simulink model "TWAICE_Cell_Model_Farasis_P75_75Ah_v8_1_3"  (R2017b)
settings: Solver=ode3  StartTime=t_start  StopTime=t_end  FixedStep=Ts  RelTol=1e-3
InitFcn:
  | m = Simulink.Mask.get(strcat(model,'/Virtual Battery Tester'));
  | cycler_selection_sel = m.getParameter('cycler_selection');
  | ts_data_repeat_tickbox_sel = m.getParameter('ts_data_repeat_tickbox');
  | if strcmp(cycler_selection_sel.Value, 'Cycle Generator')
  |      t_end = 60*60*24*365*8;
  | elseif strcmp(cycler_selection_sel.Value, 'Timeseries Data')
  |      if strcmp(ts_data_repeat_tickbox_sel.Value, 'off')
  |           t_end = Data.Time(end);
  |      elseif strcmp(ts_data_repeat_tickbox_sel.Value, 'on')
  |            t_end = 60*60*24*365*8;
  |      end
  | end
StartFcn:
  | m = Simulink.Mask.get(strcat(model,'/Virtual Battery Tester'));
  | cycler_selection_sel = m.getParameter('cycler_selection');
  | ts_data_repeat_tickbox_sel = m.getParameter('ts_data_repeat_tickbox');
  | if strcmp(cycler_selection_sel.Value, 'Cycle Generator')
  |      t_end = 60*60*24*365*8;
  | elseif strcmp(cycler_selection_sel.Value, 'Timeseries Data')
  |      if strcmp(ts_data_repeat_tickbox_sel.Value, 'off')
  |           t_end = Data.Time(end);
  |      elseif strcmp(ts_data_repeat_tickbox_sel.Value, 'on')
  |            t_end = 60*60*24*365*8;
  |      end
  | end
model workspace (MAT data in the model file):
  SOC_init = 1
values from neighbouring files (symbols this model uses):
  act = 1    [RunMe_TWAICE_Cell_Model_Farasis_P75_75Ah_v8_1_3.m]
  I_chlim = []    [RunMe_TWAICE_Cell_Model_Farasis_P75_75Ah_v8_1_3.m]
  I_dislim = []    [RunMe_TWAICE_Cell_Model_Farasis_P75_75Ah_v8_1_3.m]
  lic_no = fin_convert(Prod_lic)    [RunMe_TWAICE_Cell_Model_Farasis_P75_75Ah_v8_1_3.m]
  model = 'TWAICE_Cell_Model_Farasis_P75_75Ah_v8_1_3'    [RunMe_TWAICE_Cell_Model_Farasis_P75_75Ah_v8_1_3.m]
  soc_chlim = chargelim.Var2(inx_soc:end)'    [RunMe_TWAICE_Cell_Model_Farasis_P75_75Ah_v8_1_3.m]
  soc_dislim = dischargelim.Var2(inx_soc:end)'    [RunMe_TWAICE_Cell_Model_Farasis_P75_75Ah_v8_1_3.m]
  T_chlim = []    [RunMe_TWAICE_Cell_Model_Farasis_P75_75Ah_v8_1_3.m]
  T_dislim = []    [RunMe_TWAICE_Cell_Model_Farasis_P75_75Ah_v8_1_3.m]
  Ts = 1    [RunMe_TWAICE_Cell_Model_Farasis_P75_75Ah_v8_1_3.m]
undefined symbols (not defined in the file or in its folder): Data, T_init
libraries: simulink x3
(part 1 of 2)
settings Model: Creator=ga56rex  LastModifiedBy=MATLAB-Compute2
settings DataIOCC: LimitDataPoints=on  SaveFormat=StructureWithTime  ReturnWorkspaceOutputs=on
settings OptimizationCC: BlockReduction=off  BooleanDataType=off
settings DebuggingCC: ReadBeforeWriteMsg=DisableAll  WriteAfterWriteMsg=DisableAll  WriteAfterReadMsg=DisableAll  AlgebraicLoopMsg=error  SaveWithParameterizedLinksMsg=none  InheritedTsInSrcMsg=none  AllowSymbolicDim=off  StrictBusMsg=ErrorOnBusTreatedAsVector  SFUnexpectedBacktrackingDiag=warning  SFNoUnconditionalDefaultTransitionDiag=warning  SFExecutionAtInitializationDiag=none
settings HardwareCC: ProdBitPerPointer=32  ProdBitPerSizeT=32  ProdBitPerPtrDiffT=32  ProdLargestAtomicFloat=None  ProdIntDivRoundTo=Undefined  ProdEndianess=Unspecified  ProdWordSize=32  ProdHWDeviceType=32-bit Generic  TargetBitPerPointer=64  TargetBitPerSizeT=64  TargetBitPerPtrDiffT=64  TargetLongLongMode=on  TargetIntDivRoundTo=Zero  TargetEndianess=LittleEndian  TargetWordSize=64  TargetHWDeviceType=MATLAB Host  ProdEqTarget=off
settings ModelReferenceCC: PropagateSignalLabelsOutOfModel=off  SupportModelReferenceSimTargetCustomCode=on
settings SFSimCC: SimUserLibraries=LexActivator.lib  SimParseCustomCode=off
settings SFSimCC: SimCustomHeaderCode=|
  | #include "LexActivator.h"
  | #include "LexStatusCodes.h"
settings RTWCC: SystemTargetFile=rtwsfcn.tlc  TemplateMakefile=rtwsfcn_default_tmf  Description=S-Function Target  RTWUseSimCustomCode=on  CustomLibrary=LexActivator.lib
settings RTWCC: CustomHeaderCode=|
  | #include "LexActivator.h"
  | #include "LexStatusCodes.h"
settings CodeAppCC: StateflowObjectComments=on
settings STFCustomTargetCC: ModelReferenceCompliant=off  CompOptLevelCompliant=on  MATLABClassNameForMDSCustomization=Simulink.SoftwareTarget.TargetSpecificTriggerConfigurationBase  SystemTargetFile=rtwsfcn.tlc
settings ConfigComp: CovMetricSettings=dw  CovSaveCumulativeToWorkspaceVar=on  CovSaveSingleToWorkspaceVar=on  CovExternalEMLEnable=off  CovSFcnEnable=off

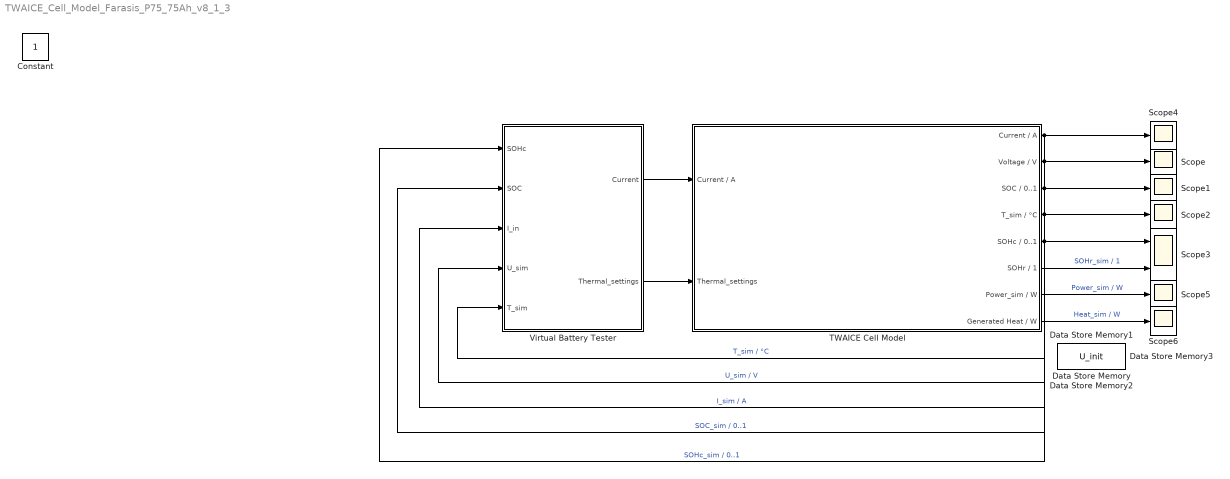
== system TWAICE_Cell_Model_Farasis_P75_75Ah_v8_1_3 ==
  Data Store Memory : DataStoreMemory  DataStoreName=SOHc_init  ReadBeforeWriteMsg=warning  WriteAfterWriteMsg=warning  WriteAfterReadMsg=warning  ShowAdditionalParam=off
  Data Store Memory1 : DataStoreMemory  DataStoreName=SOC_init  ReadBeforeWriteMsg=warning  WriteAfterWriteMsg=warning  WriteAfterReadMsg=warning  ShowAdditionalParam=off
  Data Store Memory2 : DataStoreMemory  DataStoreName=T_init  ReadBeforeWriteMsg=warning  WriteAfterWriteMsg=warning  WriteAfterReadMsg=warning  ShowAdditionalParam=off
  Data Store Memory3 : DataStoreMemory  DataStoreName=U_init  ReadBeforeWriteMsg=warning  WriteAfterWriteMsg=warning  WriteAfterReadMsg=warning  ShowAdditionalParam=off
  Scope{,1..2,4..6} (6 alike) : Scope
  Scope3 : Scope  NumInputPorts=2
  TWAICE Cell Model : Subsystem  mask{SOHc_init=1.0, SOHr_init=1.0, T_init=25, SOC_init=0.5}
      mask prompts: SOHc_init "SOHc / 0..1"; SOHr_init "SOHr / 1"; T_init "T_cell / °C"; SOC_init "SOC / 0..1"
      mask init:
      | %set_param('TWAICE_Cell_Model_MANUFACTURER_CELLTYPE_v4_2_open/TWAICE CELL MODEL','backgroundcolor','[1 0 1]')
      mask DialogControl Control4 Prompt: Electric-Thermal-Aging Model
      mask DialogControl DescTextVar Prompt: Setting Initial Parameters for the Model
      mask DialogControl Container11 Prompt: Aging
      mask DialogControl Container13 Prompt: Electric and Thermal
      mask Display: image('config/TwaiceCellModel.png'); % Use "Edit Image" on toolstrip to change.
  Virtual Battery Tester : Subsystem  mask{cycler_selection=Cycle Generator, trigger_current_ch=on, value_profile_ch=50, trigger_power_ch=off, value_charge_pause=60, discharge_type=Constant, trigger_current_dis=on, value_profile_dis=75, trigger_power_dis=off, value_discharge_pause=60, trigger_depth_dis_soc=on, value_depth_dis_soc=0, trigger_depth_dis_U=off, value_depth_dis_U=3, trigger_cv_discharge=off, value_cv_discharge_stop=0, trigger_depth_ch_soc=on, value_depth_ch_soc=1, trigger_depth_ch_U=off, value_depth_ch_U=4.2, trigger_cv_charge=off, value_cv_charge_stop=0, trigger_custom_part_resting=off, value_resting_soc=0.3, value_repeating_cycles=1, value_resting_time=20000, T_amb_set=25, stop_parameter=Equivalent Full Cycles / -, stop_value=50, start_condition=Charge, default_thermal_settings_cycgen=Use default fitted parameters, value_htc_cycgen=NaN, value_Pcool_cycgen=NaN, ts_data_profile_selection=Current / A, ts_data_repeat_tickbox=off, stop_parameter_ts_data=SOHc / 1...0, stop_value_ts_data=0.8, default_thermal_settings_ts_data=Use default fitted parameters, value_htc_ts_data=NaN, value_Pcool_ts_data=NaN, controller_tickbox=off, ctrl_type=SOC / 0...1, lower_bound_voltage=2.2, upper_bound_voltage=4.5, lower_bound_soc=0, upper_bound_soc=1, violation_trigger=off, trigger_chargelim=off, trigger_dischargelim=off}
      mask prompts: trigger_current_ch "Current / A"; value_profile_ch "Constant"; trigger_power_ch "Power / W"; value_charge_pause "Pause After Charge / s"; trigger_current_dis "Current / A"; value_profile_dis "Constant"; trigger_power_dis "Power / W"; value_discharge_pause "Pause After Discharge / s"; trigger_depth_dis_soc "SOC / 0...1"; value_depth_dis_soc "0 to 1"; trigger_depth_dis_U "Voltage / V"; trigger_cv_discharge "CV Cutoff Current Discharge/ A"; trigger_depth_ch_soc "SOC / 0...1"; value_depth_ch_soc "0 to 1"; trigger_depth_ch_U "Voltage / V"; trigger_cv_charge "CV Cutoff Current Charge / A"; trigger_custom_part_resting "Enable rest at defined SOC during cycling"; value_resting_soc "Resting SOC / 0...1"; value_repeating_cycles "Number of repeating cycles / -"; value_resting_time "Resting time / s"; ts_data_profile_selection "Input Profile"; ts_data_repeat_tickbox "Repeat timeseries data input and apply manually selected stop criteria."; controller_tickbox "Apply global cell limits"; ctrl_type "Type"; lower_bound_voltage "Global minimum voltage / V"; upper_bound_voltage "Global maximum voltage / V"; lower_bound_soc "Lower boundary SOC / 0...1"; upper_bound_soc "Upper boundary SOC / 0...1"; violation_trigger "Stop simulation upon violation (for unchecked box simulation continues with current set to zero outside the specified boundaries)"; trigger_chargelim "Enable current limitation during charging"; trigger_dischargelim "Enable current limitation during discharging"
      mask init:
      | if start_condition == 1
      |     u1_init = 0;
      | elseif start_condition == 2
      |     u1_init = 3;
      | end
      | 
      | %% Current or Power Charging
      | m = Simulink.Mask.get(gcb);
      | box_A = get_param(gcb, 'trigger_current_ch');
      | box_B = m.getParameter('trigger_power_ch');
      | if strcmp(box_A, 'off') &&  strcmp(box_B, 'off')
      |     u1_init = 10;
      | end
      mask Help:
      | This Tool generates a synthetic Power/Current Profile within specified Voltage or SOC Boundaries.
      | 
      | Box Profile Charge: Either current or power. Ticking both applies a current profile as default value.
      | 
      | Box Profile Discharge: Either current or power. Ticking both applies a current profile as default value.
      | 
      | Profile from Workspace: uses user profile in discharge direction. Must be loaded to workspace in format timeseries and named "Data_Discharge". Make sure the Data is not cleared at simulation start or reloaded into workspace. Timeseries Data must consist of the time and current/power data. Generate with: Data_Discharge = timeseries(Data, time);
      | 
      | Cycle Depth: Stop Charge/Discharge either at specified SOC or Voltage. Ticking both uses SOC as default value. SOC ranges from 0 to 1. CV phase only possible when specifying Voltage as Stop Criteria.
      | 
      | Start Condition: Charge or Discharge.
      | 
      | Stop Condition: EFC, Cycles, Time or SOHc (Capacity)
      mask TypeOptions cycler_selection: Cycle Generator | Timeseries Data
      mask Callback cycler_selection:
      | %%
      | % Enable Disable Cycle Generator and Timeseries Data Tab
      | % Block to be used modular
      | %msk_vbt = Simulink.Mask.get(strcat(model,'/Virtual Battery Tester'));
      | msk_vbt = Simulink.Mask.get(gcb);
      | for i = 1:length(msk_vbt.Parameters)
      |     names_vbt_mask{i,1} = msk_vbt.Parameters(i).Name;
      | end
      | 
      | % Block only here used
      | box_tickbox = get_param(gcb, 'cycler_selection');
      | inx_cyclegenerator_block_start = find(contains(names_vbt_mask,...
      |         'trigger_current_ch'));
      | inx_cyclegenerator_custom_part_resting = find(contains(names_vbt_mask,...
      |         'trigger_custom_part_resting'));
      | inx_cyclegenerator_T_amb = find(contains(names_vbt_mask,...
      |         'T_amb_set'));
      | inx_cyclegenerator_default_thermal_settings = find(contains(names_vbt_mask,...
      |         'default_thermal_settings_cycgen'));
      | 
      | 
      | inx_timeseriesdata_block_start = find(contains(names_vbt_mask,...
      |         'ts_data_profile_selection'));
      | inx_timeseriesdata_stop_criteria = find(contains(names_vbt_mask,...
      |         'ts_data_repeat_tickbox'));
      | inx_timeseriesdata_default_thermal_settings_ts_data = find(contains(names_vbt_mask,...
      |         'default_thermal_settings_ts_data'));
      | inx_batterycontroller_block_start = find(contains(names_vbt_mask,...
      |         'controller_tickbox'));
      | 
      | if strcmp(box_tickbox, 'Cycle Generator')
      |     % Enable Cycle Generator Block from Start to Enable Resting SOC
      |     for i_mask = inx_cyclegenerator_block_start:inx_cyclegenerator_custom_part_resting
      |         msk_vbt.Parameters(1,i_mask).Enabled = 'on';
      |     end
      |     for i_mask = inx_cyclegenerator_T_amb:inx_cyclegenerator_default_thermal_settings
      |         % Enable Cycle Generator Block from T_ambient to Radio Button
      |         % Default Thermal Setting but Default values yet as disabled
      |         msk_vbt.Parameters(1,i_mask).Enabled = 'on';
      |     end
      |     % Disable Timeseries Data Block
      |     for i_mask = inx_timeseriesdata_block_start:inx_batterycontroller_block_start-1
      |         msk_vbt.Parameters(1,i_mask).Enabled = 'off';
      |     end
      |     msk_vbt.Parameters(1,inx_timeseriesdata_stop_criteria).Value = 'off'; % Set TS Data Stop Criteria to Off (in addition to disabled)
      |     msk_vbt.Parameters(1,inx_timeseriesdata_default_thermal_settings_ts_data).Value = 'Use default fitted parameters'; % Set Thermal Parameters Ts Data to Default (in addition to disabled)
      | elseif strcmp(box_tickbox, 'Timeseries Data')
      |     for i_mask = inx_cyclegenerator_block_start:inx_timeseriesdata_block_start-1
      |         % Disable Cycle Generator Block
      |         msk_vbt.Parameters(1,i_mask).Enabled = 'off';
      |     end
      |     msk_vbt.Parameters(1,inx_cyclegenerator_custom_part_resting).Value = 'off'; % Set Enable Resting to Off (in addition to disabled)
      |     msk_vbt.Parameters(1,inx_cyclegenerator_default_thermal_settings).Value = 'Use default fitted parameters'; % Set Thermal Parameters Cyc Gen to Default (in addition to disabled)
      | 
      |     for i_mask = inx_timeseriesdata_block_start:inx_timeseriesdata_stop_criteria
      |         % Enable Timeseries Data Block
      |         msk_vbt.Parameters(1,i_mask).Enabled = 'on';
      |     end
      |     for i_mask = inx_timeseriesdata_default_thermal_settings_ts_data
      |         % Enable Timeseries Data Block
      |         msk_vbt.Parameters(1,i_mask).Enabled = 'on';
      |     end
      | end
      mask Callback trigger_current_ch:
      | %% Current or Power Charging
      | m = Simulink.Mask.get(gcb);
      | box_A = get_param(gcb, 'trigger_current_ch');
      | box_B = m.getParameter('trigger_power_ch');
      | if strcmp(box_A, 'on')
      |     box_B.Value = 'off';
      | end
      mask Callback trigger_power_ch:
      | %% Current or Power Charging
      | m = Simulink.Mask.get(gcb);
      | box_A = m.getParameter( 'trigger_current_ch');
      | box_B = get_param(gcb, 'trigger_power_ch');
      | if strcmp(box_B, 'on')
      |     box_A.Value = 'off';
      | end
      mask TypeOptions discharge_type: Constant | Profile from Workspace (Name in Workspace: Data_Discharge)
      mask Callback discharge_type:
      | m = Simulink.Mask.get(gcb);
      | dis_type = m.getParameter('discharge_type');
      | box_dis_value = m.getParameter('value_profile_dis');
      | if strcmp(dis_type.Value, 'Profile from Workspace (Name in Workspace: Data_Discharge)')
      |     box_dis_value.Enabled = 'off';
      | elseif strcmp(dis_type.Value, 'Constant')
      |     box_dis_value.Enabled = 'on';
      | end
      mask Callback trigger_current_dis:
      | %% Current or Power Discharging
      | m = Simulink.Mask.get(gcb);
      | box_A = get_param(gcb, 'trigger_current_dis');
      | box_B = m.getParameter('trigger_power_dis');
      | if strcmp(box_A, 'on')
      |     box_B.Value = 'off';
      | end
      mask Callback trigger_power_dis:
      | %% Current or Power Charging
      | m = Simulink.Mask.get(gcb);
      | box_A = m.getParameter( 'trigger_current_dis');
      | box_B = get_param(gcb, 'trigger_power_dis');
      | if strcmp(box_B, 'on')
      |     box_A.Value = 'off';
      | end
      mask Callback trigger_depth_dis_soc:
      | m = Simulink.Mask.get(gcb);
      | box_soc = get_param(gcb, 'trigger_depth_dis_soc');
      | box_U = m.getParameter('trigger_depth_dis_U');
      | box_CV = m.getParameter('trigger_cv_discharge');
      | box_CVvalue = m.getParameter('value_cv_discharge_stop');
      | if strcmp(box_soc, 'on')
      |     box_U.Value = 'off';
      |     box_CV.Value = 'off';
      |     box_CV.Enabled = 'off';
      |     box_CVvalue.Enabled = 'off';
      | end
      mask Callback trigger_depth_dis_U:
      | m = Simulink.Mask.get(gcb);
      | box_soc = m.getParameter( 'trigger_depth_dis_soc');
      | box_U = get_param(gcb,'trigger_depth_dis_U');
      | box_CV = m.getParameter('trigger_cv_discharge');
      | box_CVvalue = m.getParameter('value_cv_discharge_stop');
      | if strcmp(box_U, 'on')
      |     box_soc.Value = 'off';
      |     box_CVvalue.Enabled = 'on';
      |     box_CV.Enabled = 'on';
      | end
      mask Callback trigger_depth_ch_soc:
      | m = Simulink.Mask.get(gcb);
      | box_soc = get_param(gcb, 'trigger_depth_ch_soc');
      | box_U = m.getParameter('trigger_depth_ch_U');
      | box_CV = m.getParameter('trigger_cv_charge');
      | box_CVvalue = m.getParameter('value_cv_charge_stop');
      | if strcmp(box_soc, 'on')
      |     box_U.Value = 'off';
      |     box_CV.Value = 'off';
      |     box_CV.Enabled = 'off';
      |     box_CVvalue.Enabled = 'off';
      | end
      mask Callback trigger_depth_ch_U:
      | m = Simulink.Mask.get(gcb);
      | box_soc = m.getParameter( 'trigger_depth_ch_soc');
      | box_U = get_param(gcb,'trigger_depth_ch_U');
      | box_CV = m.getParameter('trigger_cv_charge');
      | box_CVvalue = m.getParameter('value_cv_charge_stop');
      | if strcmp(box_U, 'on')
      |     box_soc.Value = 'off';
      |     box_CVvalue.Enabled = 'on';
      |     box_CV.Enabled = 'on';
      | end
      mask Callback trigger_custom_part_resting:
      | %% Current or Power Charging
      | m = Simulink.Mask.get(gcb);
      | tickbox_custom_part_fluence = get_param(gcb, 'trigger_custom_part_resting');
      | box_rep_cycles = m.getParameter('value_repeating_cycles');
      | box_rest_time = m.getParameter('value_resting_time');
      | box_rest_soc = m.getParameter('value_resting_soc');
      | if strcmp(tickbox_custom_part_fluence, 'off')
      |     box_rep_cycles.Enabled = 'off';
      |     box_rest_time.Enabled = 'off';
      |     box_rest_soc.Enabled = 'off';
      | elseif strcmp(tickbox_custom_part_fluence, 'on')
      |     box_rep_cycles.Enabled = 'on';
      |     box_rest_time.Enabled = 'on';
      |     box_rest_soc.Enabled = 'on';
      | end
      mask TypeOptions stop_parameter: Equivalent Full Cycles / - | Cycles / - | Time / h | SOHc / 1...0
      mask TypeOptions start_condition: Charge | Discharge
      mask TypeOptions default_thermal_settings_cycgen: Use default fitted parameters | Use own adjustable parameters
      mask Callback default_thermal_settings_cycgen:
      | % Enable Disable Thermal Parameter Usage Cycle Generator
      | % Block to be used modular
      | msk_thermal_set_cycgen = Simulink.Mask.get(gcb);
      | for i = 1:length(msk_thermal_set_cycgen.Parameters)
      |     names_vbt_mask{i,1} = msk_thermal_set_cycgen.Parameters(i).Name;
      | end
      | 
      | inx_thermal_setting_cyc_generator_start = find(contains(names_vbt_mask,...
      |         'value_htc_cycgen'));
      | inx_thermal_setting_cyc_generator_end = find(contains(names_vbt_mask,...
      |         'value_Pcool_cycgen'));
      | box_thermalsetings_cycgen = get_param(gcb, 'default_thermal_settings_cycgen');
      | 
      | if strcmp(box_thermalsetings_cycgen, 'Use default fitted parameters')
      |     for i_mask = inx_thermal_setting_cyc_generator_start:inx_thermal_setting_cyc_generator_end
      |         % Disable adjustable parameters
      |         msk_thermal_set_cycgen.Parameters(1,i_mask).Enabled = 'off';
      |     end
      | elseif strcmp(box_thermalsetings_cycgen, 'Use own adjustable parameters')
      |     for i_mask = inx_thermal_setting_cyc_generator_start:inx_thermal_setting_cyc_generator_end
      |         % Enable adjustable parameters
      |         msk_thermal_set_cycgen.Parameters(1,i_mask).Enabled = 'on';
      |     end
      | end
      mask TypeOptions ts_data_profile_selection: Current / A | Power / W
      mask Callback ts_data_repeat_tickbox:
      | m = Simulink.Mask.get(gcb);
      | box_tickbox = get_param(gcb, 'ts_data_repeat_tickbox');
      | box_stop = m.getParameter('stop_parameter_ts_data');
      | box_stop2 = m.getParameter('stop_value_ts_data');
      | if strcmp(box_tickbox, 'on')
      |     box_stop.Enabled = 'on';
      |     box_stop2.Enabled = 'on';
      | end
      | if strcmp(box_tickbox, 'off')
      |     box_stop.Enabled = 'off';
      |     box_stop2.Enabled = 'off';
      | end
      mask TypeOptions stop_parameter_ts_data: Equivalent Full Cycles / - | Time / h | SOHc / 1...0
      mask TypeOptions default_thermal_settings_ts_data: Use default fitted parameters | Use own adjustable parameters
      mask Callback default_thermal_settings_ts_data:
      | % Enable Disable Thermal Parameter Usage Timeseries Data
      | % Block to be used modular
      | msk_thermal_set_ts_data = Simulink.Mask.get(gcb);
      | for i = 1:length(msk_thermal_set_ts_data.Parameters)
      |     names_vbt_mask{i,1} = msk_thermal_set_ts_data.Parameters(i).Name;
      | end
      | 
      | inx_thermal_setting_ts_data_start = find(contains(names_vbt_mask,...
      |         'value_htc_ts_data'));
      | inx_thermal_setting_ts_data_end = find(contains(names_vbt_mask,...
      |         'value_Pcool_ts_data'));
      | box_thermalsetings_ts_data = get_param(gcb, 'default_thermal_settings_ts_data');
      | 
      | if strcmp(box_thermalsetings_ts_data, 'Use default fitted parameters')
      |     for i_mask = inx_thermal_setting_ts_data_start:inx_thermal_setting_ts_data_end
      |         % Disable adjustable parameters
      |         msk_thermal_set_ts_data.Parameters(1,i_mask).Enabled = 'off';
      |     end
      | elseif strcmp(box_thermalsetings_ts_data, 'Use own adjustable parameters')
      |     for i_mask = inx_thermal_setting_ts_data_start:inx_thermal_setting_ts_data_end
      |         % Enable adjustable parameters
      |         msk_thermal_set_ts_data.Parameters(1,i_mask).Enabled = 'on';
      |     end
      | end
      mask Callback controller_tickbox:
      | m = Simulink.Mask.get(gcb);
      | box_controller = get_param(gcb, 'controller_tickbox');
      | box_1 = m.getParameter('ctrl_type');
      | box_2 = m.getParameter('lower_bound_voltage');
      | box_3 = m.getParameter('upper_bound_voltage');
      | box_4 = m.getParameter('lower_bound_soc');
      | box_5 = m.getParameter('upper_bound_soc');
      | box_6 = m.getParameter('violation_trigger');
      | box_7 = m.getParameter('trigger_chargelim');
      | box_8 = m.getParameter('trigger_dischargelim');
      | if strcmp(box_controller, 'off')
      |     box_1.Enabled = 'off';
      |     box_2.Enabled = 'off';
      |     box_3.Enabled = 'off';
      |     box_4.Enabled = 'off';
      |     box_5.Enabled = 'off';
      |     box_6.Enabled = 'off';
      |     box_7.Enabled = 'off';
      |     box_8.Enabled = 'off';
      | elseif strcmp(box_controller, 'on')
      |     box_1.Enabled = 'on';
      |     box_2.Enabled = 'on';
      |     box_3.Enabled = 'on';
      |     box_4.Enabled = 'on';
      |     box_5.Enabled = 'on';
      |     box_6.Enabled = 'on';
      |     box_7.Enabled = 'on';
      |     box_8.Enabled = 'on';
      | end
      mask TypeOptions ctrl_type: Voltage / V | SOC / 0...1
      mask Callback ctrl_type:
      | %% Current or Power Charging
      | m = Simulink.Mask.get(gcb);
      | box_type = get_param(gcb, 'ctrl_type');
      | box_min_voltage = m.getParameter( 'lower_bound_voltage');
      | box_max_voltage = m.getParameter( 'upper_bound_voltage');
      | box_min_soc = m.getParameter('lower_bound_soc');
      | box_max_soc = m.getParameter( 'upper_bound_soc');
      | 
      | if strcmp(box_type, 'Voltage / V')
      |      box_min_soc.Enabled = 'off';
      |      box_max_soc.Enabled = 'off';
      |      box_min_voltage.Enabled = 'on';
      |      box_max_voltage.Enabled = 'on';
      |  elseif strcmp(box_type, 'SOC / 0...1')
      |     box_min_soc.Enabled = 'on';
      |     box_max_soc.Enabled = 'on';
      |     box_min_voltage.Enabled = 'off';
      |     box_max_voltage.Enabled = 'off';
      |  end
      mask DialogControl Control7 Prompt: With this interface virtual battery testing is performed. Either a cycle generator can be used to generate synthetic profiles consisting of constant charge and discharge conditions within specified limits. Alternatively, timeseries data (current or power and ambient temperature) from the MATLAB workspace can be used as input into the TWAICE cell model
      mask DialogControl Container39 Prompt: Main Selection
      mask DialogControl Control41 Prompt: Use only Cycle Generator OR Timeseries Data. Please do not use both.
      mask DialogControl Control42 Prompt: Please select one of the following:
      mask DialogControl cyc_gen_container Prompt: Cycle Generator
      mask DialogControl Current_Power Prompt: Cycle Generator Options
      mask DialogControl Control38 Prompt: With the cycle generator virtual charge, discharge cycles with constant conditions can be selected.
      mask DialogControl Control39 Prompt: The constant current or power values and the upper and lower boundaries can be selected.
      mask DialogControl ChargeProfile Prompt: Charge
      mask DialogControl DischargeProfile Prompt: Discharge
      mask DialogControl Control23 Prompt: For discharge a constant value or timeseries data from the workspace can be used.
      mask DialogControl Control24 Prompt: The discharge data must be named Data_Discharge in the MATLAB workspace with the following format:
      mask DialogControl Control28 Prompt: Data_Discharge = timeseries(I, t) or Data_Discharge = timeseries(P, t) with
      mask DialogControl Control25 Prompt: - Time t in seconds
      mask DialogControl Control26 Prompt: - Current I in Ampere or Power P in W
      mask DialogControl Cycle_Depth Prompt: Cycle Depth
      mask DialogControl DischargeProfile_copy Prompt: Stop Discharge At
      mask DialogControl ChargeDepth Prompt: Stop Charge At
      mask DialogControl Rest_phase_extension Prompt: Rest at defined SOC during cycling
      mask DialogControl Control47 Prompt: With this feature, resting phases can be introduced during cycling. Before each pause, the cell will be charged to and hold at a resting SOC. At the end of the pause, the cell will be charged to the defined upper limit. Tunable parameters are:
      mask DialogControl Control48 Prompt: - Resting SOC: SOC, at which the cell should be held. Resting SOC must be above the discharge stop condition.
      mask DialogControl Control49 Prompt: - Number of repeating cycles: number of cycles to be repeated before going into the resting phase.
      mask DialogControl Control50 Prompt: - Resting time: duration of the resting period in seconds before charging to the upper limit.
      mask DialogControl Control15 Prompt: Ambient Temperature /  °C
      mask DialogControl Container10 Prompt: Start and Stop Condition
      mask DialogControl Container17 Prompt: Stop Condition
      mask DialogControl Container14 Prompt: Start Condition
      mask DialogControl Container43 Prompt: Thermal settings Cycle Generator
      mask DialogControl txt_htc Prompt: Convective heat transfer coefficient / W/(Km^2)
      mask DialogControl txt_Pcool Prompt: Cooling (>0) or heating (<0) power / W
      mask DialogControl ts_data_container Prompt: Timeseries Data
      mask DialogControl Container42 Prompt: Timeseries Data Options
      mask DialogControl Control16 Prompt: With this option the cell behaviour is simulated for timeseries data from the workspace.
      mask DialogControl Control17 Prompt: The data must be named Data in the MATLAB workspace with the following format:
      mask DialogControl Control19 Prompt: Data = timeseries([I, T_amb] , t) or Data = timeseries([P, T_amb], t) with
      mask DialogControl Control20 Prompt: - Time t in seconds.
      mask DialogControl Control21 Prompt: - Current I in Ampere or Power P in Watt.
      mask DialogControl Control31 Prompt: - Ambient Temperature T_amb in °C.
      mask DialogControl Container10_copy Prompt: Stop Condition
      mask DialogControl Control33 Prompt: By default the simulation stops once the input timeseries data ends.
      mask DialogControl Control34 Prompt: Alternatively, in this section it can be selected to repeat the input data until reaching a user defined stop criteria.
      mask DialogControl Container_ts_data Prompt: Stop Condition
      mask DialogControl Container44 Prompt: Thermal settings Timeseries Data
      mask DialogControl txt_htc_ts_data Prompt: Convective heat transfer coefficient / W/(Km^2)
      mask DialogControl txt_Pcool_ts_data Prompt: Cooling (>0) or heating (<0) power / W
      mask DialogControl Container38 Prompt: Battery Controller
      mask DialogControl Control8 Prompt: With this Controller, global voltage, SOC and temperature limits can be specified. Outside these specified boundaries the current is automatically set to zero. This battery controller can be enabled for both options (Cycle Generator and Timeseries Data).
      mask DialogControl Container31 Prompt: Global SOC/voltage limits
      mask DialogControl Control10 Prompt: Reaching those limits the current is set to zero or the simulation stopped depending on user selection.
      mask DialogControl Container32 Prompt: Current limits in dependency of temperature and SOC
      mask DialogControl Control13 Prompt: Enable maximum current limits as function of cell temperature and SOC. These can be entered seperately for charging and discharging in the excel:
      mask DialogControl Control14 Prompt: T_SOC_based_CurrentLimits.xlsx
      mask DialogControl Control14 Callback: winopen('./config/T_SOC_based_CurrentLimits.xlsx')
      mask DialogControl Control37 Prompt: Info: After changes, excel must be saved and RunMe file must be re-run to load in the latest changes into the MATLAB workspace.
      mask Display: image('config/VirtualBatteryTester.PNG'); % Use "Edit Image" on toolstrip to change.
  Constant : Constant  IOType=siggen
  wires:
  TWAICE Cell Model/3(SOC / 0..1) -> Virtual Battery Tester/2(SOC), Scope1/1  "SOC_sim / 0..1"
  TWAICE Cell Model/8(Generated Heat / W) -> Scope6/1  "Heat_sim / W"
  TWAICE Cell Model/7(Power_sim / W) -> Scope5/1  "Power_sim / W"
  TWAICE Cell Model/2(Voltage / V) -> Virtual Battery Tester/4(U_sim), Scope/1  "U_sim / V"
  TWAICE Cell Model/1(Current / A) -> Scope4/1, Virtual Battery Tester/3(I_in)  "I_sim / A"
  TWAICE Cell Model/4(T_sim / °C) -> Virtual Battery Tester/5(T_sim), Scope2/1  "T_sim / °C"
  TWAICE Cell Model/5(SOHc / 0..1) -> Virtual Battery Tester/1(SOHc), Scope3/1  "SOHc_sim / 0..1"
  TWAICE Cell Model/6(SOHr / 1) -> Scope3/2  "SOHr_sim / 1"
  Virtual Battery Tester/1(Current) -> TWAICE Cell Model/1("Current / A ")
  Virtual Battery Tester/2(Thermal_settings) -> TWAICE Cell Model/2(Thermal_settings)

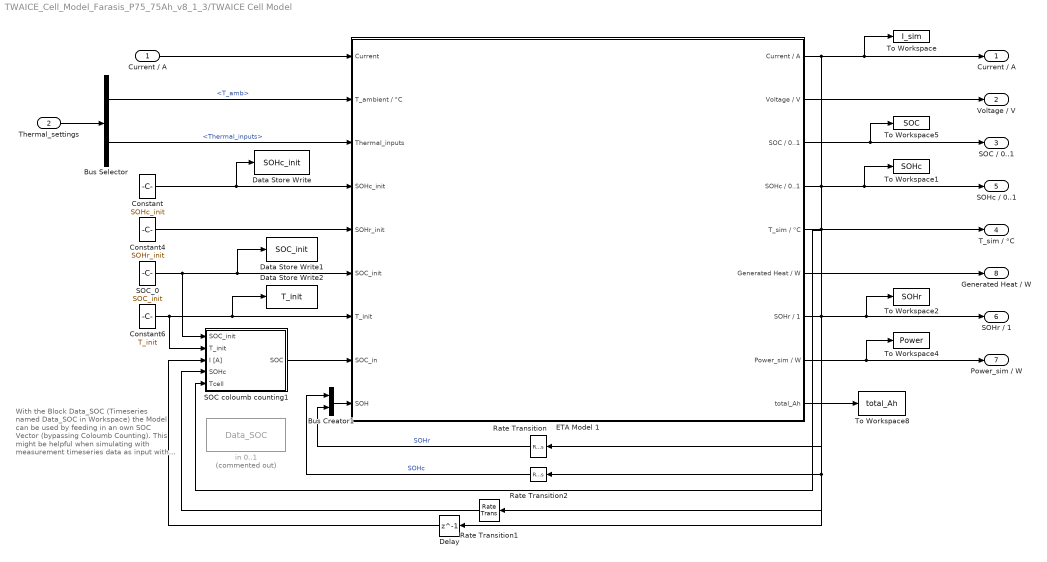
== system TWAICE_Cell_Model_Farasis_P75_75Ah_v8_1_3/TWAICE Cell Model ==
  note: With the Block Data_SOC (Timeseries named Data_SOC in Workspace)  the Model can be used by feeding in an own SOC Vector (bypassing Coloumb Counting). This might be helpful when simulating with measurement timeseries data as input with a strong SOC drift during coloumb counting.
      | For this the Block Data_SOC is to be uncommented and connected with the input SOC_in into the ETA Model.
  "Current / A " : Inport  OutDataTypeStr=double  PortDimensions=1
  Thermal_settings : Inport  Port=2
  Bus Creator1 : BusCreator  Inputs=2
  Bus Selector : BusSelector  OutputSignals=T_amb,Thermal_inputs
  Constant : Constant  Value=SOHc_init
  Constant4 : Constant  Value=SOHr_init
  Constant6 : Constant  Value=T_init
  Data Store Write : DataStoreWrite  DataStoreName=SOHc_init
  Data Store Write1 : DataStoreWrite  DataStoreName=SOC_init
  Data Store Write2 : DataStoreWrite  DataStoreName=T_init
  Delay : Delay  DelayLength=1
  ETA Model 1 : Subsystem  mask{sfcnParam1=Ts, sfcnParam2=act, sfcnParam3=lic_no}
      mask prompts: sfcnParam1 "Ts:"; sfcnParam2 "act:"; sfcnParam3 "lic_no:"
      mask help: Simulink:masks:GenSFuncDesc_MD
      mask Help: eval('feval(''rtwprivate'',''rtwhelpview'',''rtw_sfcn_block'')');
  Rate Transition : RateTransition  InitialCondition=SOHr_init
  Rate Transition1 : RateTransition  InitialCondition=SOHc_init
  Rate Transition2 : RateTransition  InitialCondition=SOHc_init
  SOC coloumb counting1 : Subsystem  mask{sfcnParam1=Ts}
      mask prompts: sfcnParam1 "Ts:"
      mask help: Simulink:masks:GenSFuncDesc_MD
      mask Help: eval('feval(''rtwprivate'',''rtwhelpview'',''rtw_sfcn_block'')');
  SOC_0 : Constant  Value=SOC_init
  To Workspace : ToWorkspace  VariableName=I_sim  SaveFormat=Timeseries  SampleTime=-1
  To Workspace1 : ToWorkspace  VariableName=SOHc  SaveFormat=Timeseries  SampleTime=-1
  To Workspace2 : ToWorkspace  VariableName=SOHr  SaveFormat=Timeseries  SampleTime=-1
  To Workspace4 : ToWorkspace  VariableName=Power  SaveFormat=Timeseries  SampleTime=-1
  To Workspace5 : ToWorkspace  VariableName=SOC  SaveFormat=Timeseries  SampleTime=-1
  To Workspace8 : ToWorkspace  VariableName=total_Ah  SaveFormat=Timeseries  SampleTime=-1
  in 0..1 : FromWorkspace  Commented=on  VariableName=Data_SOC  SampleTime=Ts  OutputAfterFinalValue=Setting to zero
  Current / A : Outport  OutDataTypeStr=double  PortDimensions=1  VectorParamsAs1DForOutWhenUnconnected=on
  Voltage / V : Outport  Port=2  OutDataTypeStr=double  PortDimensions=1  VectorParamsAs1DForOutWhenUnconnected=on
  SOC / 0..1 : Outport  Port=3  OutDataTypeStr=double  PortDimensions=1  VectorParamsAs1DForOutWhenUnconnected=on
  T_sim / °C : Outport  Port=4  OutDataTypeStr=double  PortDimensions=1  VectorParamsAs1DForOutWhenUnconnected=on
  SOHc / 0..1 : Outport  Port=5  OutDataTypeStr=double  PortDimensions=1  VectorParamsAs1DForOutWhenUnconnected=on
  SOHr / 1 : Outport  Port=6  OutDataTypeStr=double  PortDimensions=1  VectorParamsAs1DForOutWhenUnconnected=on
  Power_sim / W : Outport  Port=7  OutDataTypeStr=double  PortDimensions=1  VectorParamsAs1DForOutWhenUnconnected=on
  Generated Heat / W : Outport  Port=8  OutDataTypeStr=double  PortDimensions=1  VectorParamsAs1DForOutWhenUnconnected=on
  wires:
  "Current / A "/1 -> ETA Model 1/1("Current ")
  ETA Model 1/1(Current / A) -> Delay/1, To Workspace/1, Current / A/1
  ETA Model 1/2(Voltage / V) -> Voltage / V/1
  ETA Model 1/3(SOC / 0..1) -> SOC / 0..1/1, To Workspace5/1
  ETA Model 1/4(SOHc / 0..1) -> Rate Transition2/1, Rate Transition1/1, To Workspace1/1, SOHc / 0..1/1
  ETA Model 1/5(T_sim / °C) -> SOC coloumb counting1/5(Tcell), T_sim / °C/1
  ETA Model 1/6(Generated Heat / W) -> Generated Heat / W/1
  ETA Model 1/7(SOHr / 1) -> Rate Transition/1, To Workspace2/1, SOHr / 1/1
  ETA Model 1/8(Power_sim / W) -> To Workspace4/1, Power_sim / W/1
  Constant/1 -> ETA Model 1/4(SOHc_init), Data Store Write/1
  SOC_0/1 -> SOC coloumb counting1/1(SOC_init), ETA Model 1/6(SOC_init), Data Store Write1/1
  Constant6/1 -> SOC coloumb counting1/2(T_init), ETA Model 1/7(T_init), Data Store Write2/1
  ETA Model 1/9(total_Ah) -> To Workspace8/1
  Rate Transition1/1 -> SOC coloumb counting1/4(SOHc)
  Bus Selector/1 -> ETA Model 1/2(T_ambient / °C)  "<T_amb>"
  Thermal_settings/1 -> Bus Selector/1
  Bus Selector/2 -> ETA Model 1/3(Thermal_inputs)  "<Thermal_inputs>"
  Constant4/1 -> ETA Model 1/5(SOHr_init)
  Delay/1 -> SOC coloumb counting1/3(I [A])
  Bus Creator1/1 -> ETA Model 1/9(SOH)
  Rate Transition/1 -> Bus Creator1/2  "SOHr"
  Rate Transition2/1 -> Bus Creator1/1  "SOHc"
  SOC coloumb counting1/1(SOC) -> ETA Model 1/8(SOC_in)

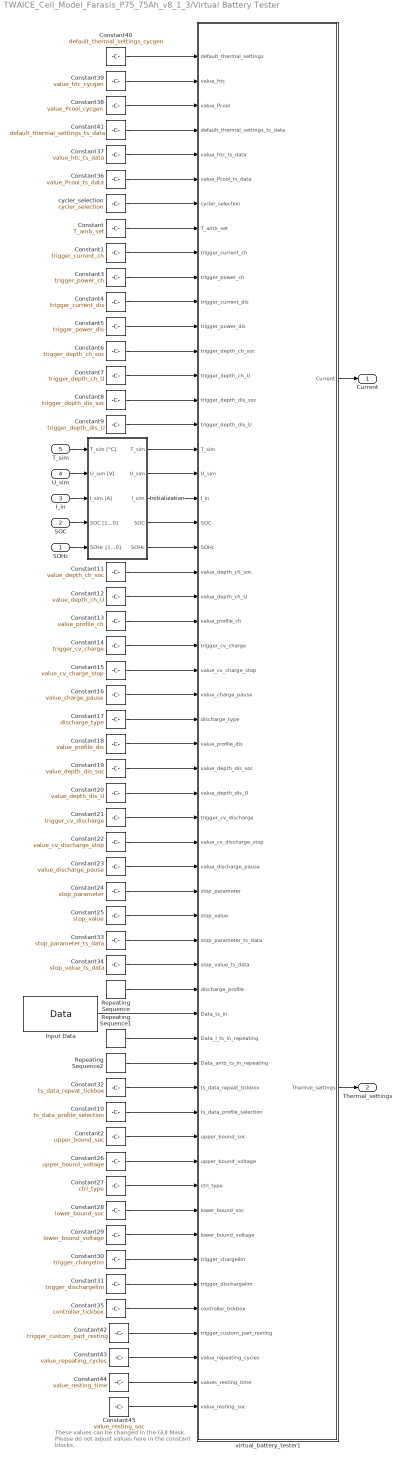
== system TWAICE_Cell_Model_Farasis_P75_75Ah_v8_1_3/Virtual Battery Tester ==
  note: These values can be changed in the GUI Mask.
      | Please do not adjust values here in the
      | constant blocks.
  SOHc : Inport
  SOC : Inport  Port=2
  I_in : Inport  Port=3
  U_sim : Inport  Port=4
  T_sim : Inport  Port=5
  Constant : Constant  Value=T_amb_set
  Constant1 : Constant  Value=trigger_current_ch
  Constant10 : Constant  Value=ts_data_profile_selection
  Constant11 : Constant  Value=value_depth_ch_soc
  Constant12 : Constant  Value=value_depth_ch_U
  Constant13 : Constant  Value=value_profile_ch
  Constant14 : Constant  Value=trigger_cv_charge
  Constant15 : Constant  Value=value_cv_charge_stop
  Constant16 : Constant  Value=value_charge_pause
  Constant17 : Constant  Value=discharge_type
  Constant18 : Constant  Value=value_profile_dis
  Constant19 : Constant  Value=value_depth_dis_soc
  Constant2 : Constant  Value=upper_bound_soc
  Constant20 : Constant  Value=value_depth_dis_U
  Constant21 : Constant  Value=trigger_cv_discharge
  Constant22 : Constant  Value=value_cv_discharge_stop
  Constant23 : Constant  Value=value_discharge_pause
  Constant24 : Constant  Value=stop_parameter
  Constant25 : Constant  Value=stop_value
  Constant26 : Constant  Value=upper_bound_voltage
  Constant27 : Constant  Value=ctrl_type
  Constant28 : Constant  Value=lower_bound_soc
  Constant29 : Constant  Value=lower_bound_voltage
  Constant3 : Constant  Value=trigger_power_ch
  Constant30 : Constant  Value=trigger_chargelim
  Constant31 : Constant  Value=trigger_dischargelim
  Constant32 : Constant  Value=ts_data_repeat_tickbox
  Constant33 : Constant  Value=stop_parameter_ts_data
  Constant34 : Constant  Value=stop_value_ts_data
  Constant35 : Constant  Value=controller_tickbox
  Constant36 : Constant  Value=value_Pcool_ts_data
  Constant37 : Constant  Value=value_htc_ts_data
  Constant38 : Constant  Value=value_Pcool_cycgen
  Constant39 : Constant  Value=value_htc_cycgen
  Constant4 : Constant  Value=trigger_current_dis
  Constant40 : Constant  Value=default_thermal_settings_cycgen
  Constant41 : Constant  Value=default_thermal_settings_ts_data
  Constant42 : Constant  Value=trigger_custom_part_resting
  Constant43 : Constant  Value=value_repeating_cycles
  Constant44 : Constant  Value=value_resting_time
  Constant45 : Constant  Value=value_resting_soc
  Constant5 : Constant  Value=trigger_power_dis
  Constant6 : Constant  Value=trigger_depth_ch_soc
  Constant7 : Constant  Value=trigger_depth_ch_U
  Constant8 : Constant  Value=trigger_depth_dis_soc
  Constant9 : Constant  Value=trigger_depth_dis_U
  Initialization : Subsystem
  Input Data : FromWorkspace  VariableName=Data  OutputAfterFinalValue=Setting to zero
  Repeating Sequence : simulink/Sources/Repeating Sequence  rep_seq_t=Data_Discharge.Time  rep_seq_y=Data_Discharge.Data
  Repeating Sequence1 : simulink/Sources/Repeating Sequence  rep_seq_t=Data.Time  rep_seq_y=Data.Data(:,1)
  Repeating Sequence2 : simulink/Sources/Repeating Sequence  rep_seq_t=Data.Time  rep_seq_y=Data.Data(:,2)
  cycler_selection : Constant  Value=cycler_selection
  virtual_battery_tester1 : Subsystem  mask{sfcnParam1=I_chlim, sfcnParam2=I_dislim, sfcnParam3=T_chlim, sfcnParam4=T_dislim, sfcnParam5=act, sfcnParam6=lic_no, sfcnParam7=soc_chlim, sfcnParam8=soc_dislim}
      mask prompts: sfcnParam1 "I_chlim:"; sfcnParam2 "I_dislim:"; sfcnParam3 "T_chlim:"; sfcnParam4 "T_dislim:"; sfcnParam5 "act:"; sfcnParam6 "lic_no:"; sfcnParam7 "soc_chlim:"; sfcnParam8 "soc_dislim:"
      mask help: Simulink:masks:GenSFuncDesc_MD
      mask Help: eval('feval(''rtwprivate'',''rtwhelpview'',''rtw_sfcn_block'')');
  Current : Outport  VectorParamsAs1DForOutWhenUnconnected=on
  Thermal_settings : Outport  Port=2  VectorParamsAs1DForOutWhenUnconnected=on
  wires:
  Constant/1 -> virtual_battery_tester1/8(T_amb_set)
  Constant1/1 -> virtual_battery_tester1/9(trigger_current_ch)
  Constant3/1 -> virtual_battery_tester1/10(trigger_power_ch)
  Constant4/1 -> virtual_battery_tester1/11(trigger_current_dis)
  Constant5/1 -> virtual_battery_tester1/12(trigger_power_dis)
  Constant6/1 -> virtual_battery_tester1/13(trigger_depth_ch_soc)
  Constant7/1 -> virtual_battery_tester1/14(trigger_depth_ch_U)
  Constant8/1 -> virtual_battery_tester1/15(trigger_depth_dis_soc)
  Constant9/1 -> virtual_battery_tester1/16(trigger_depth_dis_U)
  Constant11/1 -> virtual_battery_tester1/22(value_depth_ch_soc)
  Constant12/1 -> virtual_battery_tester1/23(value_depth_ch_U)
  Constant13/1 -> virtual_battery_tester1/24(value_profile_ch)
  Constant14/1 -> virtual_battery_tester1/25(trigger_cv_charge)
  Constant15/1 -> virtual_battery_tester1/26(value_cv_charge_stop)
  Constant16/1 -> virtual_battery_tester1/27(value_charge_pause)
  Constant17/1 -> virtual_battery_tester1/28(discharge_type)
  Constant18/1 -> virtual_battery_tester1/29(value_profile_dis)
  Constant19/1 -> virtual_battery_tester1/30(value_depth_dis_soc)
  Constant20/1 -> virtual_battery_tester1/31(value_depth_dis_U)
  Constant21/1 -> virtual_battery_tester1/32(trigger_cv_discharge)
  Constant22/1 -> virtual_battery_tester1/33(value_cv_discharge_stop)
  Constant23/1 -> virtual_battery_tester1/34(value_discharge_pause)
  Constant24/1 -> virtual_battery_tester1/35(stop_parameter)
  Constant25/1 -> virtual_battery_tester1/36(stop_value)
  Repeating Sequence/1 -> virtual_battery_tester1/39(discharge_profile)
  cycler_selection/1 -> virtual_battery_tester1/7(cycler_selection)
  Input Data/1 -> virtual_battery_tester1/40(Data_ts_in)
  Constant31/1 -> virtual_battery_tester1/51(trigger_dischargelim)
  Constant27/1 -> virtual_battery_tester1/47(ctrl_type)
  Constant30/1 -> virtual_battery_tester1/50(trigger_chargelim)
  Constant26/1 -> virtual_battery_tester1/46(upper_bound_voltage)
  Constant29/1 -> virtual_battery_tester1/49(lower_bound_voltage)
  Constant28/1 -> virtual_battery_tester1/48(lower_bound_soc)
  Constant2/1 -> virtual_battery_tester1/45(upper_bound_soc)
  virtual_battery_tester1/2(Thermal_settings) -> Thermal_settings/1
  virtual_battery_tester1/1(Current) -> Current/1
  Constant10/1 -> virtual_battery_tester1/44(ts_data_profile_selection)
  Repeating Sequence1/1 -> virtual_battery_tester1/41(Data_I_ts_in_repeating)
  Repeating Sequence2/1 -> virtual_battery_tester1/42(Data_amb_ts_in_repeating)
  Constant32/1 -> virtual_battery_tester1/43(ts_data_repeat_tickbox)
  Constant33/1 -> virtual_battery_tester1/37(stop_parameter_ts_data)
  Constant34/1 -> virtual_battery_tester1/38(stop_value_ts_data)
  Constant35/1 -> virtual_battery_tester1/52(controller_tickbox)
  T_sim/1 -> Initialization/1(T_sim [°C])
  U_sim/1 -> Initialization/2(U_sim [V])
  SOC/1 -> Initialization/4(SOC [1...0])
  I_in/1 -> Initialization/3(I_sim [A])
  SOHc/1 -> Initialization/5(SOHc [1...0])
  Initialization/1(T_sim) -> virtual_battery_tester1/17(T_sim)
  Initialization/2(U_sim) -> virtual_battery_tester1/18(U_sim)
  Initialization/3(I_sim) -> virtual_battery_tester1/19(I_in)
  Initialization/4(SOC) -> virtual_battery_tester1/20(SOC)
  Initialization/5(SOHc) -> virtual_battery_tester1/21(SOHc)
  Constant37/1 -> virtual_battery_tester1/5(value_htc_ts_data)
  Constant36/1 -> virtual_battery_tester1/6(value_Pcool_ts_data)
  Constant39/1 -> virtual_battery_tester1/2(value_htc)
  Constant38/1 -> virtual_battery_tester1/3(value_Pcool)
  Constant40/1 -> virtual_battery_tester1/1(default_thermal_settings)
  Constant41/1 -> virtual_battery_tester1/4(default_thermal_settings_ts_data)
  Constant44/1 -> virtual_battery_tester1/55(values_resting_time)
  Constant45/1 -> virtual_battery_tester1/56(value_resting_soc)
  Constant42/1 -> virtual_battery_tester1/53(trigger_custom_part_resting)
  Constant43/1 -> virtual_battery_tester1/54(value_repeating_cycles)
